simulink model "motor"  (R2024a)
settings: Solver=VariableStepAuto  StartTime=0.0  StopTime=0.8  RelTol=1e-3
undefined symbols (not defined in the file): Im, Km, Kw, Ra, Te
settings Model: Creator=115-07  LastModifiedBy=mbondarenko
settings DebuggingCC: UnconnectedInputMsg=warning  UnconnectedOutputMsg=warning  UnconnectedLineMsg=warning
settings ModelReferenceCC: EnableRefExpFcnMdlSchedulingChecks=on
settings RTWCC: GPUComputeCapability=3.5  DLArmComputeVersion=19.05

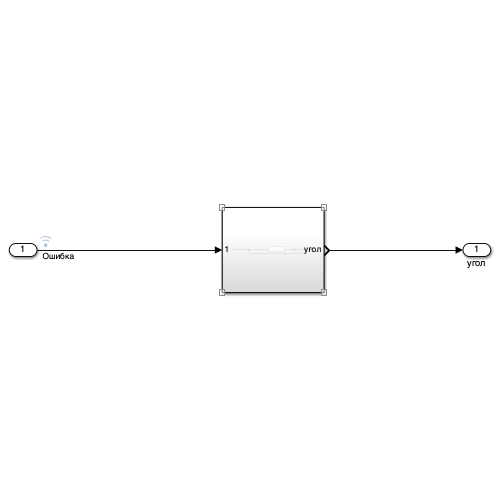
[thumbnail: Simulink's stored preview of the top-level diagram]
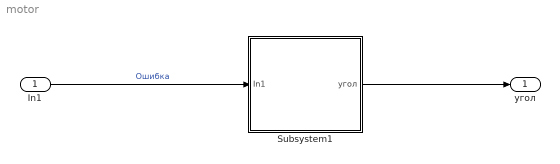
== system motor ==
  In1 : Inport
  Subsystem1 : Subsystem
  угол : Outport
  wires:
  In1/1 -> Subsystem1/1(In1)  "Ошибка"
  Subsystem1/1(угол) -> угол/1

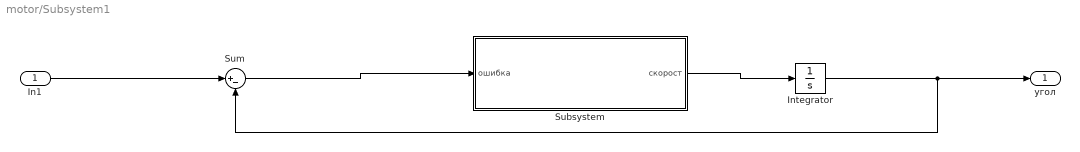
== system motor/Subsystem1 ==
  In1 : Inport
  Integrator : Integrator
  Subsystem : Subsystem
  Sum : Sum  Inputs=|+-
  угол : Outport
  wires:
  Subsystem/1(скорост) -> Integrator/1
  In1/1 -> Sum/1
  Sum/1 -> Subsystem/1(ошибка)
  Integrator/1 -> угол/1, Sum/2

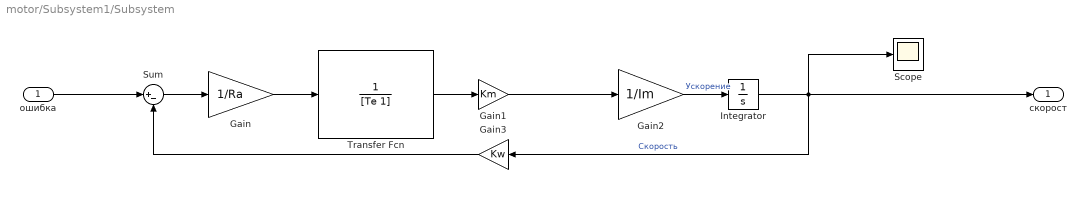
== system motor/Subsystem1/Subsystem ==
  ошибка : Inport
  Gain : Gain  Gain=1/Ra
  Gain1 : Gain  Gain=Km
  Gain2 : Gain  Gain=1/Im
  Gain3 : Gain  Gain=Kw
  Integrator : Integrator
  Scope : Scope
  Sum : Sum  Inputs=|+-
  Transfer Fcn : TransferFcn  Denominator=[Te 1]
  скорост : Outport
  wires:
  Gain1/1 -> Gain2/1
  ошибка/1 -> Sum/1
  Transfer Fcn/1 -> Gain1/1
  Integrator/1 -> скорост/1, Scope/1, Gain3/1  "Скорость"
  Gain/1 -> Transfer Fcn/1
  Gain2/1 -> Integrator/1  "Ускорение"
  Sum/1 -> Gain/1
  Gain3/1 -> Sum/2
